simulink model "HIL_Testing_SW_amantest"  (Simulink 7.5)
settings: Solver=ode1  StartTime=0.0  StopTime=Inf  FixedStep=0.001  RelTol=1e-3
PostLoadFcn:
  | , if any(exist('dsrtsu_mdlpostloadfcn', 'file') == [2, 3, 6]), try dsrtsu_mdlpostloadfcn('Execute', bdroot); catch fprintf('Error in PostLoadFcn (dsrtsu_mdlpostloadfcn) for model "%s":\n %s\n', bdroot, lasterr); end, end,
undefined symbols (not defined in the file): CeBSER_Cnt_NumTempAxisPts, ChargeCord, ChargeCord_Control, ChargeToSOCCurr, ChrgCurrLim, CrntSens1Fine, CS_SOCSetPt, CyclerMaxChrgPwr, CyclerMaxDschrgPwr, deltaAhr, Drive_1, Drive_10, Drive_11, Drive_12, Drive_13, Drive_14, Drive_15, Drive_16, Drive_17, Drive_18, Drive_19, Drive_2, Drive_20, Drive_21, Drive_22, Drive_23, Drive_24, Drive_25, Drive_26, Drive_27, Drive_28, Drive_29, Drive_3, Drive_30, Drive_31, Drive_32, Drive_33, Drive_34, Drive_35, Drive_36, Drive_37, Drive_38, Drive_39, Drive_4, Drive_40, Drive_41, Drive_42, Drive_43, Drive_44, Drive_45, Drive_46, Drive_47, Drive_48, Drive_49, Drive_5, Drive_50, Drive_51, Drive_6, Drive_7, Drive_8 ... (+50)
libraries: simulink x129, rtican x50, rti2211sailib x5, rti2211serlib x5, rti2202miolib x3
(part 23 of 23)

== stateflow chart LionsHeart/FeaturePresentation/Down_to_Business/DriveProfile_ModeControl/Scirpt Test ==
  state SwitchProfile
    entry:
    Step=Step+1;
    IndicatorSF = 2;
    ProfileClassIndex=GetIndex(ProfileScheduleClass,Step);
  state Corvette
    entry:
    IndicatorSF=0;
    PowerCycle=0;
    du:
    PowerCycle=0;
  state End_Suite
    entry:
    EndStep=99
    IndicatorSF=2;
    ex: EndStep=0;
    IndicatorSF=2;
  state Acadia
    entry:
    IndicatorSF=0;
    PowerCycle=3;
    du:
    PowerCycle=3;
  state ATS
    entry:
    IndicatorSF=0;
    PowerCycle=1;
    du:
    PowerCycle=1;
  state PowerPulse_Discharge
    entry:
    Wait=0;
    IndicatorSF=5;
    Direction =2;
    du:
    Wait=Wait+sim_step_time;
  state start
    entry:
    SuiteStep=0;
    EndStep=0;
    IndicatorSF=2;
  state Return
  state OneHundredTen_V_Charge
    entry:
    IndicatorSF = 1;
    ChargeCurrSelect=0;
    during: ChargeCurrSelect=0;
  state RestTimer
    entry:
    IndicatorSF = 2;
    RestTime = 0;
    du:
    RestTime = RestTime+sim_step_time;
  state PowerPulse_Charge
    entry:
    IndicatorSF=5;
    Direction =1;
    Wait=0;
    du:
    Wait=Wait+sim_step_time;
  state Yukon
    entry:
    IndicatorSF=0;
    PowerCycle=51;
    du:
    PowerCycle=51;
  state TwoHundredTwenty_V_Charge
    entry:
    IndicatorSF = 1;
    ChargeCurrSelect=1;
    during: ChargeCurrSelect=1;
  state XTS
    entry:
    IndicatorSF=0;
    PowerCycle=50;
    du:
    PowerCycle=50;
  state Charge_To_SOC
    entry:
    IndicatorSF = 1;
    ChargeCurrSelect=2;
    during: ChargeCurrSelect=2;
  state Reset_SOC_and_Ahr
    entry:
    IndicatorSF = 2;
    ResetSOC=1;
    ResetWaitTime=0;
    during: ResetSOC=1;
    ResetWaitTime=ResetWaitTime+sim_step_time;
    exit: ResetSOC=0;
  state Determine_Charge_Type
    entry:
    IndicatorSF = 1;
    ProfileTypeIndex=GetIndex(ProfileScheduleType,Step);
  state Determine_Drive_Type
    entry:
    IndicatorSF = 0;
    ProfileTypeIndex=GetIndex(ProfileScheduleType,Step);
  state Determine_PowerPulse_Type
    entry:
    IndicatorSF = 1;
    ProfileTypeIndex=GetIndex(ProfileScheduleType,Step);
  state Verano
    entry:
    IndicatorSF=0;
    PowerCycle=49;
    du:
    PowerCycle=49;
  state Apply_SOC_Target
    entry:
    ProfileParameter = GetIndex(ProfileScheduleParameter,Step);
    SOCTarget = ProfileParameter/100;
  state Determine_Rest_Time
    entry:
    ProfileParameter = GetIndex(ProfileScheduleParameter,Step);
  state Apply_RestTimeIn
    entry:
    RestTimeTarget = RestTimeIn;
  state Apply_ProfileParameter
    entry:
    RestTimeTarget = ProfileParameter;
  state SwitchSuite
    entry:
    SuiteStep=SuiteStep+1;
    EndStep=2;
    Step=0;
    RepeatIndex = 0;
    IndicatorSF = 2;
    SuiteIndex=GetSuiteIndex(SuiteSchedule,SuiteStep);
    Suite = SuiteIndex;
  state PrimePack_Suite
    entry:
    ProfileScheduleClass = PrimePackClass;
    ProfileScheduleType = PrimePackType;
    ProfileScheduleParameter = PrimePackParameter;
  state Use_Profile_Builder
    entry:
    ProfileScheduleClass = ProfileScheduleClassIn;
    ProfileScheduleType= ProfileScheduleTypeIn;
    ProfileScheduleParameter = ProfileScheduleParameterIn;
    ProfileScheduleParameter2 = ProfileScheduleParameterIn2;
  state Drive_With_Pulses_Suite
    entry:
    ProfileScheduleClass = DrivesWithPulsesClass;
    ProfileScheduleType = DrivesWithPulsesType;
    ProfileScheduleParameter = DrivesWithPulsesParameter;
  state End_Test
    entry:
    IndicatorSF=2;
  state Drive_To_PIC
    entry:
    ProfileScheduleClass = DriveToPICClass;
    ProfileScheduleType = DriveToPICType;
    ProfileScheduleParameter = DriveToPICParameter;
  state Aztek
    entry:
    IndicatorSF=0;
    PowerCycle=2;
    du:
    PowerCycle=2;
  state Aura
    entry:
    IndicatorSF=0;
    PowerCycle=4;
    du:
    PowerCycle=4;
  state Bel_Air
    entry:
    IndicatorSF=0;
    PowerCycle=5;
    du:
    PowerCycle=5;
  state Cruze
    entry:
    IndicatorSF=0;
    PowerCycle=6;
    du:
    PowerCycle=6;
  state Camaro
    entry:
    IndicatorSF=0;
    PowerCycle=7;
    du:
    PowerCycle=7;
  state Apply_Volt_Target1
    entry:
    ProfileParameter = GetIndex(ProfileScheduleParameter,Step);
    VoltTarget = ProfileParameter;
  state Apply_Volt_Target2
    entry:
    ProfileParameter = GetIndex(ProfileScheduleParameter,Step);
    VoltTarget = ProfileParameter;
  state Reset_Run
    entry:
    IndicatorSF = 2;
    ResetTime = 0;
    ResetRun = 1;
    du:
    ResetRun=1;
    ResetTime = ResetTime+sim_step_time;
    exit:
    ResetRun=0;
    SetChamberT_ToBatTemp = 0;
  state Determine_Reset_Time
    entry:
    ProfileParameter = GetIndex(ProfileScheduleParameter,Step);
  state Apply_DefaultTime
    entry:
    ResetTarget = 150;
  state Apply_ParameterTime
    entry:
    ResetTarget = ProfileParameter;
  state Capacity_Test
    entry:
    IndicatorSF = 3;
    du:
    IndicatorSF = 3;
  state Caprice
    entry:
    IndicatorSF=0;
    PowerCycle=8;
    du:
    PowerCycle=8;
  state Colorado
    entry:
    IndicatorSF=0;
    PowerCycle=9;
    du:
    PowerCycle=9;
  state CTSv
    entry:
    IndicatorSF=0;
    PowerCycle=10;
    du:
    PowerCycle=10;
  state Cobalt
    entry:
    IndicatorSF=0;
    PowerCycle=11;
    du:
    PowerCycle=11;
  state TimerForContactorstoClose
    entry:
    WTime=0;
    du:
    WTime=WTime+sim_step_time;
  state DTS
    entry:
    IndicatorSF=0;
    PowerCycle=12;
    du:
    PowerCycle=12;
  state El_Camino
    entry:
    IndicatorSF=0;
    PowerCycle=13;
    du:
    PowerCycle=13;
  state Equinox
    entry:
    IndicatorSF=0;
    PowerCycle=14;
    du:
    PowerCycle=14;
  state Encore
    entry:
    IndicatorSF=0;
    PowerCycle=15;
    du:
    PowerCycle=15;
  state Enclave
    entry:
    IndicatorSF=0;
    PowerCycle=16;
    du:
    PowerCycle=16;
  state OCV_Test
    entry:
    IndicatorSF = 6;
    du:
    IndicatorSF = 6;
  state ELR
    entry:
    IndicatorSF=0;
    PowerCycle=17;
    du:
    PowerCycle=17;
  state El_Dorado
    entry:
    IndicatorSF=0;
    PowerCycle=18;
    du:
    PowerCycle=18;
  state HHR
    entry:
    IndicatorSF=0;
    PowerCycle=19;
    du:
    PowerCycle=19;
  state Impala
    entry:
    IndicatorSF=0;
    PowerCycle=20;
    du:
    PowerCycle=20;
  state Lacrosse
    entry:
    IndicatorSF=0;
    PowerCycle=21;
    du:
    PowerCycle=21;
  state MontiCarlo
    entry:
    IndicatorSF=0;
    PowerCycle=22;
    du:
    PowerCycle=22;
  state Malibu
    entry:
    IndicatorSF=0;
    PowerCycle=23;
    du:
    PowerCycle=23;
  state Montana
    entry:
    IndicatorSF=0;
    PowerCycle=24;
    du:
    PowerCycle=24;
  state Nova
    entry:
    IndicatorSF=0;
    PowerCycle=25;
    du:
    PowerCycle=25;
  state Determine_Drive_Start
    entry:
    IndicatorSF = 0;
    StartTime=GetIndex(ProfileScheduleParameter,Step);
  state Determine_Drive_End
    entry:
    IndicatorSF = 0;
    EndTime=GetIndex(ProfileScheduleParameter2,Step);
  state Chevelle
    entry:
    IndicatorSF=0;
    PowerCycle=26;
    du:
    PowerCycle=26;
  state Idle_ConstPower
    entry:
    IndicatorSF =7;
    Wait =0;
    du:
    IndicatorSF = 7;
    Wait = Wait +sim_step_time;
  state Determine_Idle_ConstPower_Time
    entry:
    ProfileParameter = GetIndex(ProfileScheduleParameter,Step);
    IdleTime=ProfileParameter;
    Idle_Type = 1;
  state Determine_IdlePower
    entry:
    ProfileParameter = GetIndex(ProfileScheduleParameter2,Step);
    PowerReq=ProfileParameter;
  state Chevette
    entry:
    IndicatorSF=0;
    PowerCycle=27;
    du:
    PowerCycle=27;
  state Corvair
    entry:
    IndicatorSF=0;
    PowerCycle=28;
    du:
    PowerCycle=28;
  state GrandPrix
    entry:
    IndicatorSF=0;
    PowerCycle=29;
    du:
    PowerCycle=29;
  state G6
    entry:
    IndicatorSF=0;
    PowerCycle=30;
    du:
    PowerCycle=30;
  state Determine_RaterPulse_Type
    entry:
    IndicatorSF = 2;
    ProfileTypeIndex=GetIndex(ProfileScheduleType,Step);
  state RatePulse_Discharge
    entry:
    Wait=0;
    IndicatorSF=8;
    Direction =2;
    du:
    Wait=Wait+sim_step_time;
  state RatePulse_Charge
    entry:
    IndicatorSF=8;
    Direction =1;
    Wait=0;
    du:
    Wait=Wait+sim_step_time;
  state Determine_CurrentLimit
    entry:
    ProfileParameter = GetIndex(ProfileScheduleParameter,Step);
    CurrLim=ProfileParameter;
  state Determine_Rate
    entry:
    ProfileParameter = GetIndex(ProfileScheduleParameter2,Step);
    Rate=ProfileParameter;
  state Increment_Test
    entry:
    IndicatorSF = 9;
    du:
    IndicatorSF = 9;
  state G8
    entry:
    IndicatorSF=0;
    PowerCycle=31;
    du:
    PowerCycle=31;
  state Outlook
    entry:
    IndicatorSF=0;
    PowerCycle=32;
    du:
    PowerCycle=32;
  state Canyon
    entry:
    IndicatorSF=0;
    PowerCycle=33;
    du:
    PowerCycle=33;
  state Firebird
    entry:
    IndicatorSF=0;
    PowerCycle=34;
    du:
    PowerCycle=34;
  state Regal
    entry:
    IndicatorSF=0;
    PowerCycle=35;
    du:
    PowerCycle=35;
  state Silverado
    entry:
    IndicatorSF=0;
    PowerCycle=36;
    du:
    PowerCycle=36;
  state Sierra
    entry:
    IndicatorSF=0;
    PowerCycle=37;
    du:
    PowerCycle=37;
  state Sonic
    entry:
    IndicatorSF=0;
    PowerCycle=38;
    du:
    PowerCycle=38;
  state Spark
    entry:
    IndicatorSF=0;
    PowerCycle=39;
    du:
    PowerCycle=39;
  state Sky
    entry:
    IndicatorSF=0;
    PowerCycle=40;
    du:
    PowerCycle=40;
  state Solstice
    entry:
    IndicatorSF=0;
    PowerCycle=41;
    du:
    PowerCycle=41;
  state SRX
    entry:
    IndicatorSF=0;
    PowerCycle=42;
    du:
    PowerCycle=42;
  state Escalade
    entry:
    IndicatorSF=0;
    PowerCycle=43;
    du:
    PowerCycle=43;
  state Terrain
    entry:
    IndicatorSF=0;
    PowerCycle=44;
    du:
    PowerCycle=44;
  state Torrent
    entry:
    IndicatorSF=0;
    PowerCycle=45;
    du:
    PowerCycle=45;
  state TransAm
    entry:
    IndicatorSF=0;
    PowerCycle=46;
    du:
    PowerCycle=46;
  state Traverse
    entry:
    IndicatorSF=0;
    PowerCycle=47;
    du:
    PowerCycle=47;
  state Tahoe
    entry:
    IndicatorSF=0;
    PowerCycle=48;
    du:
    PowerCycle=48;
  state Determine_SetChamberT_ToBatTemp
    entry:
    ProfileParameter = GetIndex(ProfileScheduleParameter2,Step);
    SetChamberT_ToBatTemp = ProfileParameter;
  state Apply_SetChamberT_ToBatTemp
    entry:
    SetChamberT_ToBatTemp = 1;
  state Apply_DontSetChamberT_ToBatTemp
    entry:
    SetChamberT_ToBatTemp = 0;
  state Idle_ConstCurrent
    entry:
    IndicatorSF =7;
    Wait =0;
    du:
    IndicatorSF = 7;
    Wait = Wait +sim_step_time;
  state Determine_Idle_ConstCurrent_Time
    entry:
    ProfileParameter = GetIndex(ProfileScheduleParameter,Step);
    IdleTime=ProfileParameter;
    Idle_Type = 2;
  state Determine_IdleCurrent
    entry:
    ProfileParameter = GetIndex(ProfileScheduleParameter2,Step);
    CurrentReq=ProfileParameter;
  state Determine_Idle_Type
    entry:
    IndicatorSF = 1;
    ProfileTypeIndex=GetIndex(ProfileScheduleType,Step);
  state Repeat
    entry:
    IndicatorSF = 2;
    RepeatCount = GetIndex(ProfileScheduleParameter,Step);
    RepeatStep
  state RepeatEnd
    entry:
    IndicatorSF = 2;
    RepeatIndex = 0;
    Step=Step+1;
  state RepeatJumpLoop
    entry:
    IndicatorSF = 2;
    Jumps = GetIndex(ProfileScheduleParameter2,Step);
    Jumps = Jumps + 1;
    during:
    RepeatIndex = RepeatIndex+1;
    Step=1;
    RepeatStep
  SwitchProfile -> Determine_Charge_Type [order 2] : [ProfileClassIndex == 1]
  Return -> (junction 900) [order 1] : [(Run==1) && (SkipStep==0)]
  Corvette -> Return [order 2] : [(LoopTime>= ProfileEndTime) && (LoopTime>0)]
  PowerPulse_Discharge -> Return [order 2] : [(PulseStep>= 2) && (Wait>1)]
  ATS -> Return [order 2] : [(LoopTime>= ProfileEndTime) && (LoopTime>0)]
  Determine_Charge_Type -> Apply_Volt_Target2 [order 2] : [ProfileTypeIndex==2]
  (default) -> start
  Corvette -> Return [order 1] : [Run==0]
  PowerPulse_Discharge -> Return [order 1] : [Run==0]
  ATS -> Return [order 1] : [Run==0]
  start -> SwitchSuite : [ManualMode==0 && Run == 1]
  Reset_SOC_and_Ahr -> Return [order 2] : [ResetWaitTime>=2]
  End_Suite -> start [order 2] : [Run==0]
  Determine_Drive_End -> Yukon [order 52] : [ProfileTypeIndex==52]
  OneHundredTen_V_Charge -> Return [order 2] : [ChargeStep>=99]
  RestTimer -> Return [order 2] : [RestTime>=RestTimeTarget]
  Determine_Drive_End -> Corvette [order 1] : [ProfileTypeIndex == 1]
  Reset_SOC_and_Ahr -> Return [order 1] : [Run==0]
  Determine_Drive_End -> Acadia [order 4] : [ProfileTypeIndex == 4]
  RestTimer -> Return [order 1] : [Run==0]
  Acadia -> Return [order 1] : [Run==0]
  Acadia -> Return [order 2] : [(LoopTime>= ProfileEndTime) && (LoopTime>0)]
  Determine_Charge_Type -> Apply_SOC_Target [order 3] : [ProfileTypeIndex==3]
  Determine_Charge_Type -> Apply_Volt_Target1 [order 1] : [ProfileTypeIndex==1]
  PowerPulse_Charge -> Return [order 2] : [(PulseStep>= 2) && (Wait>1)]
  Determine_Drive_End -> XTS [order 51] : [ProfileTypeIndex==51]
  SwitchProfile -> End_Suite [order 13] : [ProfileClassIndex==0]
  PowerPulse_Charge -> Return [order 1] : [Run==0]
  TwoHundredTwenty_V_Charge -> Return [order 2] : [ChargeStep>=99]
  TwoHundredTwenty_V_Charge -> Return [order 1] : [Run==0]
  Determine_Drive_End -> Tahoe [order 49] : [ProfileTypeIndex==49]
  Determine_Drive_End -> Traverse [order 48] : [ProfileTypeIndex==48]
  Determine_Drive_End -> ATS [order 2] : [ProfileTypeIndex == 2]
  SwitchProfile -> start [order 1] : [Run==0]
  OneHundredTen_V_Charge -> Return [order 3] : [SkipStep==1]
  TwoHundredTwenty_V_Charge -> Return [order 3] : [SkipStep==1]
  Determine_Drive_End -> TransAm [order 47] : [ProfileTypeIndex==47]
  RestTimer -> Return [order 3] : [SkipStep==1]
  Corvette -> Return [order 3] : [SkipStep==1]
  ATS -> Return [order 3] : [SkipStep==1]
  Acadia -> Return [order 3] : [SkipStep==1]
  PowerPulse_Charge -> Return [order 3] : [SkipStep==1]
  Determine_Drive_End -> Torrent [order 46] : [ProfileTypeIndex==46]
  Determine_Drive_End -> Terrain [order 45] : [ProfileTypeIndex==45]
  Determine_Drive_End -> Escalade [order 44] : [ProfileTypeIndex==44]
  Reset_SOC_and_Ahr -> Return [order 3] : [SkipStep==1]
  Charge_To_SOC -> Return [order 1] : [ChargeStep>=99]
  Charge_To_SOC -> Return [order 2] : [Run==0]
  Charge_To_SOC -> Return [order 3] : [SkipStep==1]
  Determine_Drive_End -> Verano [order 50] : [ProfileTypeIndex==50]
  SwitchProfile -> Determine_Drive_Type [order 5] : [ProfileClassIndex == 2]
  Determine_PowerPulse_Type -> PowerPulse_Discharge [order 1] : [ProfileTypeIndex == 1]
  Determine_PowerPulse_Type -> PowerPulse_Charge [order 2] : [ProfileTypeIndex == 2]
  SwitchProfile -> Determine_PowerPulse_Type [order 6] : [ProfileClassIndex == 3]
  SwitchProfile -> Determine_Rest_Time [order 10] : [ProfileClassIndex == 5]
  SwitchProfile -> Reset_SOC_and_Ahr [order 8] : [ProfileClassIndex == 4]
  Determine_Drive_End -> Spark [order 40] : [ProfileTypeIndex==40]
  Determine_Drive_End -> Sonic [order 39] : [ProfileTypeIndex==39]
  Determine_Drive_End -> Sierra [order 38] : [ProfileTypeIndex==38]
  Determine_Drive_End -> Sky [order 41] : [ProfileTypeIndex==41]
  Apply_SOC_Target -> Charge_To_SOC [order 2]
  Determine_Rest_Time -> Apply_RestTimeIn [order 1] : [ProfileParameter == 0]
  Apply_RestTimeIn -> RestTimer
  Determine_Rest_Time -> Apply_ProfileParameter [order 2] : [ProfileParameter != 0]
  Apply_ProfileParameter -> RestTimer
  SwitchSuite -> PrimePack_Suite [order 1] : [SuiteIndex == 1]
  SwitchSuite -> Use_Profile_Builder [order 4] : [SuiteIndex == 10]
  SwitchSuite -> Drive_With_Pulses_Suite [order 2] : [SuiteIndex == 2]
  PrimePack_Suite -> SwitchProfile
  Drive_With_Pulses_Suite -> SwitchProfile
  Use_Profile_Builder -> SwitchProfile
  End_Suite -> SwitchSuite [order 1] : after(1000,tick) [(Run==1) && (SkipStep==0)]
  SwitchSuite -> End_Test [order 5] : [SuiteIndex == 0]
  End_Test -> start : [Run == 0]
  SwitchSuite -> Drive_To_PIC [order 3] : [SuiteIndex == 3]
  Drive_To_PIC -> SwitchProfile
  PowerPulse_Discharge -> Return [order 3] : [SkipStep==1]
  (junction 900) -> Use_Profile_Builder [order 2] : [SuiteIndex == 10]
  (junction 900) -> SwitchProfile [order 1] : [SuiteIndex != 10]
  Aztek -> Return [order 2] : [(LoopTime>= ProfileEndTime) && (LoopTime>0)]
  Aztek -> Return [order 1] : [Run==0]
  Aztek -> Return [order 3] : [SkipStep==1]
  Determine_Drive_End -> Aztek [order 3] : [ProfileTypeIndex == 3]
  Aura -> Return [order 1] : [Run==0]
  Aura -> Return [order 2] : [(LoopTime>= ProfileEndTime) && (LoopTime>0)]
  Aura -> Return [order 3] : [SkipStep==1]
  Bel_Air -> Return [order 1] : [Run==0]
  Bel_Air -> Return [order 2] : [(LoopTime>= ProfileEndTime) && (LoopTime>0)]
  Bel_Air -> Return [order 3] : [SkipStep==1]
  Cruze -> Return [order 1] : [Run==0]
  Cruze -> Return [order 2] : [(LoopTime>= ProfileEndTime) && (LoopTime>0)]
  Cruze -> Return [order 3] : [SkipStep==1]
  Camaro -> Return [order 1] : [Run==0]
  Camaro -> Return [order 2] : [(LoopTime>= ProfileEndTime) && (LoopTime>0)]
  Camaro -> Return [order 3] : [SkipStep==1]
  Camaro -> Return [order 4] : [(EnblSOCTerm==1) && (SOC<(SOCDeplete))]
  Cruze -> Return [order 4] : [(EnblSOCTerm==1) && (SOC<(SOCDeplete))]
  Bel_Air -> Return [order 4] : [(EnblSOCTerm==1) && (SOC<(SOCDeplete))]
  Determine_Drive_End -> Aura [order 5] : [ProfileTypeIndex == 5]
  Determine_Drive_End -> Bel_Air [order 6] : [ProfileTypeIndex == 6]
  Determine_Drive_End -> Cruze [order 7] : [ProfileTypeIndex == 7]
  Determine_Drive_End -> Camaro [order 8] : [ProfileTypeIndex == 8]
  Aura -> Return [order 4] : [(EnblSOCTerm==1) && (SOC<(SOCDeplete/100))]
  Apply_SOC_Target -> Return [order 1] : [(SOCTarget > 100) || (SOCTarget < 0)]
  OneHundredTen_V_Charge -> Return [order 1] : [Run==0]
  Corvette -> Return [order 4] : [(EnblSOCTerm==1) && (SOC<(SOCDeplete))]
  ATS -> Return [order 4] : [(EnblSOCTerm==1) && (SOC<(SOCDeplete))]
  Aztek -> Return [order 4] : [(EnblSOCTerm==1) && (SOC<(SOCDeplete))]
  Acadia -> Return [order 4] : [(EnblSOCTerm==1) && (SOC<(SOCDeplete))]
  Apply_Volt_Target1 -> OneHundredTen_V_Charge
  Determine_Drive_End -> Lacrosse [order 23] : [ProfileTypeIndex == 22]
  Apply_Volt_Target2 -> TwoHundredTwenty_V_Charge
  Determine_Drive_End -> Impala [order 21] : [ProfileTypeIndex == 21]
  Reset_Run -> TimerForContactorstoClose [order 1] : [ResetTime>=ResetTarget]
  Reset_Run -> Return [order 2] : [Run==0]
  Reset_Run -> Return [order 3] : [SkipStep==1]
  Determine_Reset_Time -> Apply_DefaultTime [order 1] : [ProfileParameter == 0]
  Determine_Reset_Time -> Apply_ParameterTime [order 2] : [ProfileParameter != 0]
  Apply_DefaultTime -> Determine_SetChamberT_ToBatTemp
  Apply_ParameterTime -> Determine_SetChamberT_ToBatTemp
  SwitchProfile -> Determine_Reset_Time [order 12] : [ProfileClassIndex ==6]
  SwitchProfile -> Capacity_Test [order 7] : [ProfileClassIndex==7]
  Capacity_Test -> Return [order 3] : [SkipStep==1]
  Capacity_Test -> Return [order 2] : [CapStep==99]
  Capacity_Test -> Return [order 1] : [Run==0]
  Determine_Drive_End -> Caprice [order 9] : [ProfileTypeIndex == 9]
  Caprice -> Return [order 1] : [Run==0]
  Caprice -> Return [order 2] : [(LoopTime>= ProfileEndTime) && (LoopTime>0)]
  Caprice -> Return [order 3] : [SkipStep==1]
  Caprice -> Return [order 4] : [(EnblSOCTerm==1) && (SOC<(SOCDeplete))]
  Determine_Drive_End -> Colorado [order 10] : [ProfileTypeIndex == 10]
  Determine_Drive_End -> CTSv [order 11] : [ProfileTypeIndex == 11]
  Colorado -> Return [order 1] : [Run==0]
  Colorado -> Return [order 2] : [(LoopTime>= ProfileEndTime) && (LoopTime>0)]
  Colorado -> Return [order 3] : [SkipStep==1]
  Colorado -> Return [order 4] : [(EnblSOCTerm==1) && (SOC<(SOCDeplete))]
  CTSv -> Return [order 1] : [Run==0]
  CTSv -> Return [order 2] : [(LoopTime>= ProfileEndTime) && (LoopTime>0)]
  CTSv -> Return [order 3] : [SkipStep==1]
  CTSv -> Return [order 4] : [(EnblSOCTerm==1) && (SOC<(SOCDeplete))]
  Determine_Drive_End -> Cobalt [order 12] : [ProfileTypeIndex == 12]
  Cobalt -> Return [order 1] : [Run==0]
  Cobalt -> Return [order 2] : [(LoopTime>= ProfileEndTime) && (LoopTime>0)]
  Cobalt -> Return [order 3] : [SkipStep==1]
  Cobalt -> Return [order 4] : [(EnblSOCTerm==1) && (SOC<(SOCDeplete/100))]
  TimerForContactorstoClose -> Return [order 1] : [WTime>10]
  TimerForContactorstoClose -> Return [order 2] : [Run==0]
  TimerForContactorstoClose -> Return [order 3] : [SkipStep==1]
  Determine_Drive_End -> DTS [order 13] : [ProfileTypeIndex == 13]
  DTS -> Return [order 1] : [Run==0]
  DTS -> Return [order 2] : [(LoopTime>= ProfileEndTime) && (LoopTime>0)]
  DTS -> Return [order 3] : [SkipStep==1]
  DTS -> Return [order 4] : [(EnblSOCTerm==1) && (SOC<(SOCDeplete))]
  El_Camino -> Return [order 1] : [Run==0]
  El_Camino -> Return [order 2] : [(LoopTime>= ProfileEndTime) && (LoopTime>0)]
  El_Camino -> Return [order 3] : [SkipStep==1]
  El_Camino -> Return [order 4] : [(EnblSOCTerm==1) && (SOC<(SOCDeplete))]
  Determine_Drive_End -> El_Camino [order 14] : [ProfileTypeIndex == 14]
  Equinox -> Return [order 1] : [Run==0]
  Equinox -> Return [order 2] : [(LoopTime>= ProfileEndTime) && (LoopTime>0)]
  Equinox -> Return [order 3] : [SkipStep==1]
  Equinox -> Return [order 4] : [(EnblSOCTerm==1) && (SOC<(SOCDeplete))]
  Determine_Drive_End -> Equinox [order 15] : [ProfileTypeIndex == 15]
  Encore -> Return [order 1] : [Run==0]
  Encore -> Return [order 2] : [(LoopTime>= ProfileEndTime) && (LoopTime>0)]
  Encore -> Return [order 3] : [SkipStep==1]
  Encore -> Return [order 4] : [(EnblSOCTerm==1) && (SOC<(SOCDeplete))]
  Enclave -> Return [order 1] : [Run==0]
  Enclave -> Return [order 2] : [(LoopTime>= ProfileEndTime) && (LoopTime>0)]
  Enclave -> Return [order 3] : [SkipStep==1]
  Enclave -> Return [order 4] : [(EnblSOCTerm==1) && (SOC<(SOCDeplete))]
  Determine_Drive_End -> Encore [order 17] : [ProfileTypeIndex == 16]
  Determine_Drive_End -> Enclave [order 16] : [ProfileTypeIndex == 17]
  OCV_Test -> Return [order 3] : [SkipStep==1]
  OCV_Test -> Return [order 2] : [OCVStep==99]
  OCV_Test -> Return [order 1] : [Run==0]
  SwitchProfile -> RepeatJumpLoop [order 4] : [RepeatIndex !=0 && ProfileClassIndex==100]
  ELR -> Return [order 1] : [Run==0]
  ELR -> Return [order 2] : [(LoopTime>= ProfileEndTime) && (LoopTime>0)]
  ELR -> Return [order 3] : [SkipStep==1]
  ELR -> Return [order 4] : [(EnblSOCTerm==1) && (SOC<(SOCDeplete))]
  El_Dorado -> Return [order 1] : [Run==0]
  El_Dorado -> Return [order 2] : [(LoopTime>= ProfileEndTime) && (LoopTime>0)]
  El_Dorado -> Return [order 3] : [SkipStep==1]
  El_Dorado -> Return [order 5] : [(EnblSOCTerm==1) && (SOC<(SOCDeplete))]
  HHR -> Return [order 1] : [Run==0]
  HHR -> Return [order 2] : [(LoopTime>= ProfileEndTime) && (LoopTime>0)]
  HHR -> Return [order 4] : [SkipStep==1]
  HHR -> Return [order 5] : [(EnblSOCTerm==1) && (SOC<(SOCDeplete))]
  Impala -> Return [order 1] : [Run==0]
  Impala -> Return [order 3] : [(LoopTime>= ProfileEndTime) && (LoopTime>0)]
  Impala -> Return [order 4] : [SkipStep==1]
  Impala -> Return [order 5] : [(EnblSOCTerm==1) && (SOC<(SOCDeplete))]
  Lacrosse -> Return [order 2] : [(LoopTime>= ProfileEndTime) && (LoopTime>0)]
  Lacrosse -> Return [order 3] : [SkipStep==1]
  Lacrosse -> Return [order 4] : [(EnblSOCTerm==1) && (SOC<(SOCDeplete))]
  Lacrosse -> Return [order 1] : [Run==0]
  Determine_Drive_End -> ELR [order 18] : [ProfileTypeIndex == 18]
  Determine_Drive_End -> El_Dorado [order 19] : [ProfileTypeIndex == 19]
  Determine_Drive_End -> HHR [order 20] : [ProfileTypeIndex == 20]
  MontiCarlo -> Return [order 2] : [(LoopTime>= ProfileEndTime) && (LoopTime>0)]
  MontiCarlo -> Return [order 4] : [SkipStep==1]
  MontiCarlo -> Return [order 5] : [(EnblSOCTerm==1) && (SOC<(SOCDeplete))]
  MontiCarlo -> Return [order 1] : [Run==0]
  Malibu -> Return [order 2] : [(LoopTime>= ProfileEndTime) && (LoopTime>0)]
  Malibu -> Return [order 3] : [SkipStep==1]
  Malibu -> Return [order 4] : [(EnblSOCTerm==1) && (SOC<(SOCDeplete))]
  Malibu -> Return [order 1] : [Run==0]
  Montana -> Return [order 2] : [(LoopTime>= ProfileEndTime) && (LoopTime>0)]
  Montana -> Return [order 3] : [SkipStep==1]
  Montana -> Return [order 4] : [(EnblSOCTerm==1) && (SOC<(SOCDeplete))]
  Montana -> Return [order 1] : [Run==0]
  Nova -> Return [order 2] : [(LoopTime>= ProfileEndTime) && (LoopTime>0)]
  Nova -> Return [order 3] : [SkipStep==1]
  Nova -> Return [order 4] : [(EnblSOCTerm==1) && (SOC<(SOCDeplete))]
  RatePulse_Charge -> Return [order 4] : [(EnblSOCTerm==1) && (SOC<(SOCDeplete))]
  Determine_Drive_End -> MontiCarlo [order 22] : [ProfileTypeIndex==23]
  Determine_Drive_End -> Malibu [order 29] : [ProfileTypeIndex==24]
  Determine_Drive_End -> Montana [order 31] : [ProfileTypeIndex==25]
  Determine_Drive_End -> Nova [order 30] : [ProfileTypeIndex==26]
  Corvette -> Return [order 5] : [SwitchMode==1]
  ATS -> Return [order 5] : [SwitchMode==1]
  Aztek -> Return [order 5] : [SwitchMode==1]
  Acadia -> Return [order 5] : [SwitchMode==1]
  Aura -> Return [order 5] : [SwitchMode==1]
  Bel_Air -> Return [order 5] : [SwitchMode==1]
  Cruze -> Return [order 5] : [SwitchMode==1]
  Camaro -> Return [order 5] : [SwitchMode==1]
  Caprice -> Return [order 5] : [SwitchMode==1]
  Colorado -> Return [order 5] : [SwitchMode==1]
  CTSv -> Return [order 5] : [SwitchMode==1]
  Cobalt -> Return [order 5] : [SwitchMode==1]
  DTS -> Return [order 5] : [SwitchMode==1]
  El_Camino -> Return [order 5] : [SwitchMode==1]
  Equinox -> Return [order 5] : [SwitchMode==1]
  Encore -> Return [order 5] : [SwitchMode==1]
  Enclave -> Return [order 5] : [SwitchMode==1]
  Determine_Drive_Type -> Determine_Drive_Start
  Determine_Drive_Start -> Determine_Drive_End
  Chevelle -> Return [order 1] : [Run==0]
  Chevelle -> Return [order 2] : [(LoopTime>= ProfileEndTime) && (LoopTime>0)]
  Chevelle -> Return [order 3] : [SkipStep==1]
  Nova -> Return [order 1] : [Run==0]
  Chevelle -> Return [order 4] : [(EnblSOCTerm==1) && (SOC<(SOCDeplete))]
  Determine_Drive_End -> Chevelle [order 24] : [ProfileTypeIndex==27]
  Idle_ConstPower -> Return [order 4] : [SkipStep==1]
  Idle_ConstPower -> Return [order 3] : [(IdleStep==99) && (Wait>1)]
  Idle_ConstPower -> Return [order 1] : [Run==0]
  Apply_DontSetChamberT_ToBatTemp -> Reset_Run
  Determine_Idle_ConstPower_Time -> Determine_IdlePower [order 1] : [IdleTime!=0]
  Determine_Idle_ConstPower_Time -> Return [order 2] : [IdleTime==0]
  Idle_ConstPower -> Return [order 2] : [FA!=0]
  OneHundredTen_V_Charge -> Return [order 4] : [FA!=0]
  TwoHundredTwenty_V_Charge -> Return [order 4] : [FA!=0]
  Determine_Drive_End -> SRX [order 43] : [ProfileTypeIndex==43]
  Determine_Drive_End -> Solstice [order 42] : [ProfileTypeIndex==42]
  Charge_To_SOC -> Return [order 4] : [FA!=0]
  Determine_Drive_End -> Silverado [order 37] : [ProfileTypeIndex==37]
  Corvette -> Return [order 6] : [FA!=0]
  ATS -> Return [order 6] : [FA!=0]
  Aztek -> Return [order 6] : [FA!=0]
  Acadia -> Return [order 6] : [FA!=0]
  Aura -> Return [order 6] : [FA!=0]
  Bel_Air -> Return [order 6] : [FA!=0]
  Cruze -> Return [order 6] : [FA!=0]
  Camaro -> Return [order 6] : [FA!=0]
  Caprice -> Return [order 6] : [FA!=0]
  Colorado -> Return [order 6] : [FA!=0]
  CTSv -> Return [order 6] : [FA!=0]
  Cobalt -> Return [order 6] : [FA!=0]
  DTS -> Return [order 6] : [FA!=0]
  El_Camino -> Return [order 6] : [FA!=0]
  Equinox -> Return [order 6] : [FA!=0]
  Encore -> Return [order 6] : [FA!=0]
  Enclave -> Return [order 6] : [FA!=0]
  ELR -> Return [order 6] : [FA!=0]
  HHR -> Return [order 6] : [FA!=0]
  Impala -> Return [order 6] : [FA!=0]
  Lacrosse -> Return [order 6] : [FA!=0]
  MontiCarlo -> Return [order 6] : [FA!=0]
  Malibu -> Return [order 5] : [FA!=0]
  Montana -> Return [order 5] : [FA!=0]
  Nova -> Return [order 5] : [FA!=0]
  Chevelle -> Return [order 5] : [FA!=0]
  PowerPulse_Discharge -> Return [order 4] : [FA!=0]
  PowerPulse_Charge -> Return [order 4] : [FA!=0]
  Reset_SOC_and_Ahr -> Return [order 4] : [FA!=0]
  RestTimer -> Return [order 4] : [FA!=0]
  Capacity_Test -> Return [order 4] : [FA!=0]
  OCV_Test -> Return [order 4] : [FA!=0]
  Determine_IdlePower -> Idle_ConstPower [order 1] : [(PowerReq!=0) || (ManualIdle==1)]
  Determine_IdlePower -> Return [order 2] : [(PowerReq)==0 && (ManualIdle!=1)]
  G6 -> Return [order 5] : [FA!=0]
  Chevette -> Return [order 1] : [Run==0]
  Chevette -> Return [order 2] : [(LoopTime>= ProfileEndTime) && (LoopTime>0)]
  Chevette -> Return [order 3] : [SkipStep==1]
  Chevette -> Return [order 4] : [(EnblSOCTerm==1) && (SOC<(SOCDeplete))]
  MontiCarlo -> Return [order 3] : [SwitchMode==1]
  Determine_Drive_End -> Chevette [order 27] : [ProfileTypeIndex==28]
  Chevette -> Return [order 6] : [FA!=0]
  Determine_Drive_End -> G6 [order 25] : [ProfileTypeIndex==31]
  Corvair -> Return [order 1] : [Run==0]
  Corvair -> Return [order 2] : [(LoopTime>= ProfileEndTime) && (LoopTime>0)]
  Corvair -> Return [order 3] : [SkipStep==1]
  Corvair -> Return [order 4] : [(EnblSOCTerm==1) && (SOC<(SOCDeplete))]
  RatePulse_Discharge -> Return [order 5] : [(EnblSOCTerm==1) && (SOC<(SOCDeplete))]
  Determine_Drive_End -> Corvair [order 28] : [ProfileTypeIndex==29]
  Corvair -> Return [order 6] : [FA!=0]
  Corvair -> Return [order 5] : [SwitchMode==1]
  GrandPrix -> Return [order 1] : [Run==0]
  GrandPrix -> Return [order 2] : [(LoopTime>= ProfileEndTime) && (LoopTime>0)]
  GrandPrix -> Return [order 3] : [SkipStep==1]
  GrandPrix -> Return [order 4] : [(EnblSOCTerm==1) && (SOC<(SOCDeplete))]
  Chevette -> Return [order 5] : [SwitchMode==1]
  Determine_Drive_End -> GrandPrix [order 26] : [ProfileTypeIndex==30]
  GrandPrix -> Return [order 5] : [FA!=0]
  G6 -> Return [order 4] : [(EnblSOCTerm==1) && (SOC<(SOCDeplete))]
  G6 -> Return [order 1] : [Run==0]
  G6 -> Return [order 2] : [(LoopTime>= ProfileEndTime) && (LoopTime>0)]
  G6 -> Return [order 3] : [SkipStep==1]
  Determine_CurrentLimit -> Determine_Rate [order 1] : [CurrLim!=0]
  Determine_Rate -> Determine_RaterPulse_Type [order 1] : [Rate!=0]
  Determine_CurrentLimit -> Return [order 2] : [CurrLim==0]
  Determine_Rate -> Return [order 2] : [Rate==0]
  Determine_RaterPulse_Type -> RatePulse_Discharge [order 1] : [ProfileTypeIndex==1]
  Determine_RaterPulse_Type -> RatePulse_Charge [order 2] : [ProfileTypeIndex==2]
  RatePulse_Discharge -> Return [order 2] : [(RateStep== 2) && (Wait>1)]
  RatePulse_Discharge -> Return [order 1] : [Run==0]
  RatePulse_Discharge -> Return [order 3] : [SkipStep==1]
  RatePulse_Discharge -> Return [order 4] : [FA!=0]
  RatePulse_Charge -> Return [order 5] : [FA!=0]
  RatePulse_Charge -> Return [order 2] : [(RateStep== 2) && (Wait>1)]
  RatePulse_Charge -> Return [order 1] : [Run==0]
  RatePulse_Charge -> Return [order 3] : [SkipStep==1]
  Apply_SetChamberT_ToBatTemp -> Reset_Run
  Determine_SetChamberT_ToBatTemp -> Apply_DontSetChamberT_ToBatTemp [order 2] : [SetChamberT_ToBatTemp == 0]
  Increment_Test -> Return [order 1] : [Run==0]
  Increment_Test -> Return [order 2] : [IncrementStep==99]
  Increment_Test -> Return [order 3] : [SkipStep ==1]
  Increment_Test -> Return [order 4] : [FA!=0]
  Determine_Drive_End -> G8 [order 32] : [ProfileTypeIndex==32]
  Determine_Drive_End -> Outlook [order 33] : [ProfileTypeIndex==33]
  Determine_Drive_End -> Canyon [order 34] : [ProfileTypeIndex==34]
  Determine_Drive_End -> Firebird [order 35] : [ProfileTypeIndex==35]
  Determine_Drive_End -> Regal [order 36] : [ProfileTypeIndex==36]
  G8 -> Return [order 5] : [FA!=0]
  Lacrosse -> Return [order 5] : [SwitchMode==1]
  G8 -> Return [order 4] : [(EnblSOCTerm==1) && (SOC<(SOCDeplete))]
  G8 -> Return [order 1] : [Run==0]
  G8 -> Return [order 2] : [(LoopTime>= ProfileEndTime) && (LoopTime>0)]
  G8 -> Return [order 3] : [SkipStep==1]
  Outlook -> Return [order 5] : [FA!=0]
  Impala -> Return [order 2] : [SwitchMode==1]
  Outlook -> Return [order 4] : [(EnblSOCTerm==1) && (SOC<(SOCDeplete))]
  Outlook -> Return [order 1] : [Run==0]
  Outlook -> Return [order 2] : [(LoopTime>= ProfileEndTime) && (LoopTime>0)]
  Outlook -> Return [order 3] : [SkipStep==1]
  Canyon -> Return [order 5] : [FA!=0]
  HHR -> Return [order 3] : [SwitchMode==1]
  Canyon -> Return [order 4] : [(EnblSOCTerm==1) && (SOC<(SOCDeplete))]
  Canyon -> Return [order 1] : [Run==0]
  Canyon -> Return [order 2] : [(LoopTime>= ProfileEndTime) && (LoopTime>0)]
  Canyon -> Return [order 3] : [SkipStep==1]
  Firebird -> Return [order 6] : [FA!=0]
  El_Dorado -> Return [order 6] : [FA!=0]
  Firebird -> Return [order 4] : [(EnblSOCTerm==1) && (SOC<(SOCDeplete))]
  Firebird -> Return [order 1] : [Run==0]
  Firebird -> Return [order 2] : [(LoopTime>= ProfileEndTime) && (LoopTime>0)]
  Firebird -> Return [order 3] : [SkipStep==1]
  Regal -> Return [order 6] : [FA!=0]
  El_Dorado -> Return [order 4] : [SwitchMode==1]
  Regal -> Return [order 4] : [(EnblSOCTerm==1) && (SOC<(SOCDeplete))]
  Regal -> Return [order 1] : [Run==0]
  Regal -> Return [order 2] : [(LoopTime>= ProfileEndTime) && (LoopTime>0)]
  Regal -> Return [order 3] : [SkipStep==1]
  Silverado -> Return [order 6] : [FA!=0]
  ELR -> Return [order 5] : [SwitchMode==1]
  Silverado -> Return [order 4] : [(EnblSOCTerm==1) && (SOC<(SOCDeplete))]
  Silverado -> Return [order 1] : [Run==0]
  Silverado -> Return [order 2] : [(LoopTime>= ProfileEndTime) && (LoopTime>0)]
  Silverado -> Return [order 3] : [SkipStep==1]
  Sierra -> Return [order 5] : [FA!=0]
  Determine_Idle_Type -> Determine_Idle_ConstPower_Time [order 1] : [ProfileTypeIndex == 1]
  Sierra -> Return [order 4] : [(EnblSOCTerm==1) && (SOC<(SOCDeplete))]
  Sierra -> Return [order 1] : [Run==0]
  Sierra -> Return [order 2] : [(LoopTime>= ProfileEndTime) && (LoopTime>0)]
  Sierra -> Return [order 3] : [SkipStep==1]
  Sonic -> Return [order 5] : [FA!=0]
  Determine_Idle_Type -> Determine_Idle_ConstCurrent_Time [order 2] : [ProfileTypeIndex == 2]
  Sonic -> Return [order 4] : [(EnblSOCTerm==1) && (SOC<(SOCDeplete))]
  Sonic -> Return [order 1] : [Run==0]
  Sonic -> Return [order 2] : [(LoopTime>= ProfileEndTime) && (LoopTime>0)]
  Sonic -> Return [order 3] : [SkipStep==1]
  Spark -> Return [order 5] : [FA!=0]
  Determine_IdleCurrent -> Return [order 2] : [(CurrentReq)==0 && (ManualIdle!=1)]
  Spark -> Return [order 4] : [(EnblSOCTerm==1) && (SOC<(SOCDeplete))]
  Spark -> Return [order 1] : [Run==0]
  Spark -> Return [order 2] : [(LoopTime>= ProfileEndTime) && (LoopTime>0)]
  Spark -> Return [order 3] : [SkipStep==1]
  Sky -> Return [order 5] : [FA!=0]
  Determine_IdleCurrent -> Idle_ConstCurrent [order 1] : [(CurrentReq!=0) || (ManualIdle==1)]
  Sky -> Return [order 4] : [(EnblSOCTerm==1) && (SOC<(SOCDeplete))]
  Sky -> Return [order 1] : [Run==0]
  Sky -> Return [order 2] : [(LoopTime>= ProfileEndTime) && (LoopTime>0)]
  Sky -> Return [order 3] : [SkipStep==1]
  Solstice -> Return [order 6] : [FA!=0]
  Solstice -> Return [order 5] : [SwitchMode==1]
  Solstice -> Return [order 4] : [(EnblSOCTerm==1) && (SOC<(SOCDeplete))]
  Solstice -> Return [order 1] : [Run==0]
  Solstice -> Return [order 2] : [(LoopTime>= ProfileEndTime) && (LoopTime>0)]
  Solstice -> Return [order 3] : [SkipStep==1]
  SRX -> Return [order 6] : [FA!=0]
  SRX -> Return [order 5] : [SwitchMode==1]
  SRX -> Return [order 4] : [(EnblSOCTerm==1) && (SOC<(SOCDeplete))]
  SRX -> Return [order 1] : [Run==0]
  SRX -> Return [order 2] : [(LoopTime>= ProfileEndTime) && (LoopTime>0)]
  SRX -> Return [order 3] : [SkipStep==1]
  Escalade -> Return [order 6] : [FA!=0]
  Escalade -> Return [order 5] : [SwitchMode==1]
  Escalade -> Return [order 4] : [(EnblSOCTerm==1) && (SOC<(SOCDeplete))]
  Escalade -> Return [order 1] : [Run==0]
  Escalade -> Return [order 2] : [(LoopTime>= ProfileEndTime) && (LoopTime>0)]
  Escalade -> Return [order 3] : [SkipStep==1]
  Terrain -> Return [order 6] : [FA!=0]
  Terrain -> Return [order 5] : [SwitchMode==1]
  Terrain -> Return [order 4] : [(EnblSOCTerm==1) && (SOC<(SOCDeplete))]
  Terrain -> Return [order 1] : [Run==0]
  Terrain -> Return [order 2] : [(LoopTime>= ProfileEndTime) && (LoopTime>0)]
  Terrain -> Return [order 3] : [SkipStep==1]
  Torrent -> Return [order 6] : [FA!=0]
  Torrent -> Return [order 5] : [SwitchMode==1]
  Torrent -> Return [order 4] : [(EnblSOCTerm==1) && (SOC<(SOCDeplete))]
  Torrent -> Return [order 1] : [Run==0]
  Torrent -> Return [order 2] : [(LoopTime>= ProfileEndTime) && (LoopTime>0)]
  Torrent -> Return [order 3] : [SkipStep==1]
  TransAm -> Return [order 6] : [FA!=0]
  TransAm -> Return [order 5] : [SwitchMode==1]
  TransAm -> Return [order 4] : [(EnblSOCTerm==1) && (SOC<(SOCDeplete))]
  TransAm -> Return [order 1] : [Run==0]
  TransAm -> Return [order 2] : [(LoopTime>= ProfileEndTime) && (LoopTime>0)]
  TransAm -> Return [order 3] : [SkipStep==1]
  Traverse -> Return [order 6] : [FA!=0]
  Traverse -> Return [order 5] : [SwitchMode==1]
  Traverse -> Return [order 4] : [(EnblSOCTerm==1) && (SOC<(SOCDeplete))]
  Traverse -> Return [order 1] : [Run==0]
  Traverse -> Return [order 2] : [(LoopTime>= ProfileEndTime) && (LoopTime>0)]
  Traverse -> Return [order 3] : [SkipStep==1]
  Tahoe -> Return [order 6] : [FA!=0]
  Tahoe -> Return [order 5] : [SwitchMode==1]
  Tahoe -> Return [order 4] : [(EnblSOCTerm==1) && (SOC<(SOCDeplete))]
  Tahoe -> Return [order 1] : [Run==0]
  Tahoe -> Return [order 2] : [(LoopTime>= ProfileEndTime) && (LoopTime>0)]
  Tahoe -> Return [order 3] : [SkipStep==1]
  Verano -> Return [order 6] : [FA!=0]
  Verano -> Return [order 5] : [SwitchMode==1]
  Verano -> Return [order 4] : [(EnblSOCTerm==1) && (SOC<(SOCDeplete))]
  Verano -> Return [order 1] : [Run==0]
  Verano -> Return [order 2] : [(LoopTime>= ProfileEndTime) && (LoopTime>0)]
  Verano -> Return [order 3] : [SkipStep==1]
  XTS -> Return [order 6] : [FA!=0]
  XTS -> Return [order 5] : [SwitchMode==1]
  XTS -> Return [order 4] : [(EnblSOCTerm==1) && (SOC<(SOCDeplete))]
  XTS -> Return [order 1] : [Run==0]
  XTS -> Return [order 2] : [(LoopTime>= ProfileEndTime) && (LoopTime>0)]
  XTS -> Return [order 3] : [SkipStep==1]
  Yukon -> Return [order 6] : [FA!=0]
  Yukon -> Return [order 5] : [SwitchMode==1]
  Yukon -> Return [order 4] : [(EnblSOCTerm==1) && (SOC<(SOCDeplete))]
  Yukon -> Return [order 1] : [Run==0]
  Yukon -> Return [order 2] : [(LoopTime>= ProfileEndTime) && (LoopTime>0)]
  Yukon -> Return [order 3] : [SkipStep==1]
  Determine_SetChamberT_ToBatTemp -> Apply_SetChamberT_ToBatTemp [order 1] : [SetChamberT_ToBatTemp != 0]
  SwitchProfile -> Determine_Idle_Type [order 11] : [ProfileClassIndex==8]
  SwitchProfile -> Increment_Test [order 15] : [ProfileClassIndex == 18]
  SwitchProfile -> Determine_CurrentLimit [order 14] : [ProfileClassIndex == 10]
  SwitchProfile -> OCV_Test [order 9] : [ProfileClassIndex==9]
  Idle_ConstCurrent -> Return [order 4] : [SkipStep==1]
  Idle_ConstCurrent -> Return [order 3] : [(IdleStep==99) && (Wait>1)]
  Idle_ConstCurrent -> Return [order 1] : [Run==0]
  Determine_Idle_ConstCurrent_Time -> Determine_IdleCurrent [order 1] : [IdleTime!=0]
  Determine_Idle_ConstCurrent_Time -> Return [order 2] : [IdleTime==0]
  Idle_ConstCurrent -> Return [order 2] : [FA!=0]
  Firebird -> Return [order 5] : [SwitchMode==1]
  Regal -> Return [order 5] : [SwitchMode==1]
  Silverado -> Return [order 5] : [SwitchMode==1]
  SwitchProfile -> Repeat [order 3] : [ProfileClassIndex==100&&RepeatIndex==0]
  RepeatEnd -> SwitchProfile
  Repeat -> RepeatJumpLoop
  RepeatJumpLoop -> RepeatEnd [order 2] : [RepeatIndex == (RepeatCount+1)]
  RepeatJumpLoop -> SwitchProfile [order 1] : [RepeatIndex != (RepeatCount+1)]
  Return -> start [order 2] : [Run == 0]
  data: ProfileList function_input uint8 size=20; index function_input double; ProfileInd function_output uint8 size=1; ProfileList function_input uint8 size=20; index function_input double; ProfileInd function_output uint8 size=1; ProfileList function_input uint8 size=20; index function_input double; ProfileInd function_output uint8 size=1; ProfileList function_input uint8 size=20; index function_input double; ProfileInd function_output uint8 size=1; ProfileList function_input double size=20; index function_input double; ProfileInd function_output double size=1; ProfileList function_input double size=20; index function_input double; ProfileInd function_output double size=1; SuiteList function_input uint8 size=12; index function_input uint8; ProfileInd function_output uint8 size=1; ProfileList function_input double size=20; index function_input double; ProfileInd function_output double size=1; ProfileList function_input double size=20; index function_input double; ProfileInd function_output double size=1; ProfileList function_input double size=20; index function_input double; ProfileInd function_output double size=1; ProfileList function_input double size=20; index function_input double; ProfileInd function_output double size=1; ProfileList function_input double size=20; index function_input double; ProfileInd function_output double size=1; ProfileList function_input double size=20; index function_input double; ProfileInd function_output double size=1; ProfileList function_input double size=20; index function_input double; ProfileInd function_output double size=1; ProfileList function_input uint8 size=20; index function_input double; ProfileInd function_output uint8 size=1; ProfileList function_input double size=20; index function_input double; ProfileInd function_output double size=1; ProfileList function_input double size=20; index function_input double; ProfileInd function_output double size=1; ProfileList function_input double size=20; index function_input double; ProfileInd function_output double size=1; ProfileList function_input double size=20; index function_input double; ProfileInd function_output double size=1; ProfileList function_input double size=20; index function_input double; ProfileInd function_output double size=1; ProfileList function_input uint8 size=20; index function_input double; ProfileInd function_output uint8 size=1; Jumps local int8; RepeatCount local int8; data local double; ProfileList function_input double size=20; index function_input double; ProfileInd function_output double size=1; Jumps local int8; RepeatCount local int8; ProfileList function_input double size=20; index function_input double; ProfileInd function_output double size=1; ProfileEndTime input double; SOC input double; VoltTarget output double; PowerCycle output double; LoopTime input single; IndicatorSF output double; ChargeCurrSelect output single; ChargeStep input double; sim_step_time input double; Direction output single; PulseStep input single; ManualMode input double; RestTimeIn input double; RestTime local double; Run input boolean; SuiteSchedule input uint8 size=12; Wait local double; ProfileScheduleClassIn input uint8 size=20; i local single; ProfileClassIndex local uint8 size=1; ResetSOC output boolean; ResetWaitTime local double; ProfileScheduleTypeIn input uint8 size=20; ProfileScheduleParameterIn input double size=20; ProfileScheduleParameterIn2 input double size=20; SkipStep input boolean; ProfileTypeIndex local uint8 size=1; ProfileParameter local double; RestTimeTarget local double; SuiteStep output uint8; ProfileScheduleClass output uint8 size=20; ProfileScheduleType output uint8 size=20; ProfileScheduleParameter output double size=20; Step output single; Suite output single; SuiteIndex local uint8; PrimePackClass local uint8 size=20 =1 5 4 1 1 5 0 0 0 0 0 0 0 0 0 0 0 0 0 0; PrimePackType local uint8 size=20 =4 0 0 5 5 0 0 0 0 0 0 0 0 0 0 0 0 0 0 0; PrimePackParameter local double size=20 =0 3600 0 80 94 0 3600 0 0 0 0 0 0 0 0 0 0 0 0 0; DrivesWithPulsesClass local uint8 size=20 =2 2 3 2 3 2 0 0 0 0 0 0 0 0 0 0 0 0 0 0; DrivesWithPulsesType local uint8 size=20 =1 4 1 2 2 2 0 0 0 0 0 0 0 0 0 0 0 0 0 0; DrivesWithPulsesParameter local double size=20 =0 0 0 0 0 0 0 0 0 0 0 0 0 0 0 0 0 0 0 0; DriveToPICClass local uint8 size=20 =2 2 2 5 1 5 0 0 0 0 0 0 0 0 0 0 0 0 0 0; DriveToPICType local uint8 size=20 =1 4 2 0 1 0 0 0 0 0 0 0 0 0 0 0 0 0 0 0; DriveToPICParameter local double size=20 =0 0 0 3600 0 3600 0 0 0 0 0 0 0 0 0 0 0 0 0 0; EnblSOCTerm input boolean; SOCDeplete input single; DriveToPICClass_Init local double; DriveToPICParameter_Init local double; DriveToPICType_Init local double; DrivesWithPulsesClass_Init local double; DrivesWithPulsesParameter_Init local double; DrivesWithPulsesType_Init local double; PrimePackClass_Init local double; PrimePackParameter_Init local double; PrimePackType_Init local double; ResetTarget local double; ResetTime local double; ResetRun output double; CapStep input single; WTime local double; EndStep output double; OCVStep input single; SOCTarget output double; SwitchMode input double; StartTime output double; EndTime output double; ProfileScheduleParameter2 local double size=20; FA input double; IdleStep input double; IdleTime output double; PowerReq output double; CurrentReq output double; ManualIdle input double; Rate output single; CurrLim output double; RateStep input double; IncrementStep input double; SetChamberT_ToBatTemp output boolean; RepeatIndex local double; Idle_Type output double; RepeatStep local double; data1 local double; Jumps local double; RepeatCount local double
  function ProfileInd  = GetIndex(ProfileList,index):
    | function ProfileInd  = GetIndex(ProfileList,index)
    | 
    | ProfileInd = ProfileList(index);
    | 
    | end
  function ProfileInd  = GetIndex(ProfileList,index):
    | function ProfileInd  = GetIndex(ProfileList,index)
    | 
    | ProfileInd = ProfileList(index);
    | 
    | end
  function ProfileInd  = GetIndex(ProfileList,index):
    | function ProfileInd  = GetIndex(ProfileList,index)
    | 
    | ProfileInd = ProfileList(index);
    | 
    | end
  function ProfileInd  = GetIndex(ProfileList,index):
    | function ProfileInd  = GetIndex(ProfileList,index)
    | 
    | ProfileInd = ProfileList(index);
    | 
    | end
  function ProfileInd  = GetIndex(ProfileList,index):
    | function ProfileInd  = GetIndex(ProfileList,index)
    | 
    | ProfileInd = ProfileList(index);
    | 
    | end
  function ProfileInd  = GetIndex(ProfileList,index):
    | function ProfileInd  = GetIndex(ProfileList,index)
    | 
    | ProfileInd = ProfileList(index);
    | 
    | end
  function ProfileInd  = GetSuiteIndex(SuiteList,index):
    | function ProfileInd  = GetSuiteIndex(SuiteList,index)
    | 
    | ProfileInd = SuiteList(index);
    | 
    | end
  function ProfileInd  = GetIndex(ProfileList,index):
    | function ProfileInd  = GetIndex(ProfileList,index)
    | 
    | ProfileInd = ProfileList(index);
    | 
    | end
  function ProfileInd  = GetIndex(ProfileList,index):
    | function ProfileInd  = GetIndex(ProfileList,index)
    | 
    | ProfileInd = ProfileList(index);
    | 
    | end
  function ProfileInd  = GetIndex(ProfileList,index):
    | function ProfileInd  = GetIndex(ProfileList,index)
    | 
    | ProfileInd = ProfileList(index);
    | 
    | end
  function ProfileInd  = GetIndex(ProfileList,index):
    | function ProfileInd  = GetIndex(ProfileList,index)
    | 
    | ProfileInd = ProfileList(index);
    | 
    | end
  function ProfileInd  = GetIndex(ProfileList,index):
    | function ProfileInd  = GetIndex(ProfileList,index)
    | 
    | ProfileInd = ProfileList(index);
    | 
    | end
  function ProfileInd  = GetIndex(ProfileList,index):
    | function ProfileInd  = GetIndex(ProfileList,index)
    | 
    | ProfileInd = ProfileList(index);
    | 
    | end
  function ProfileInd  = GetIndex(ProfileList,index):
    | function ProfileInd  = GetIndex(ProfileList,index)
    | 
    | ProfileInd = ProfileList(index);
    | 
    | end
  function ProfileInd  = GetIndex(ProfileList,index):
    | function ProfileInd  = GetIndex(ProfileList,index)
    | 
    | ProfileInd = ProfileList(index);
    | 
    | end
  function ProfileInd  = GetIndex(ProfileList,index):
    | function ProfileInd  = GetIndex(ProfileList,index)
    | 
    | ProfileInd = ProfileList(index);
    | 
    | end
  function ProfileInd  = GetIndex(ProfileList,index):
    | function ProfileInd  = GetIndex(ProfileList,index)
    | 
    | ProfileInd = ProfileList(index);
    | 
    | end
  function ProfileInd  = GetIndex(ProfileList,index):
    | function ProfileInd  = GetIndex(ProfileList,index)
    | 
    | ProfileInd = ProfileList(index);
    | 
    | end
  function ProfileInd  = GetIndex(ProfileList,index):
    | function ProfileInd  = GetIndex(ProfileList,index)
    | 
    | ProfileInd = ProfileList(index);
    | 
    | end
  function ProfileInd  = GetIndex(ProfileList,index):
    | function ProfileInd  = GetIndex(ProfileList,index)
    | 
    | ProfileInd = ProfileList(index);
    | 
    | end
  function ProfileInd  = GetIndex(ProfileList,index):
    | function ProfileInd  = GetIndex(ProfileList,index)
    | 
    | ProfileInd = ProfileList(index);
    | 
    | end
  function ProfileInd  = GetIndex(ProfileList,index):
    | function ProfileInd  = GetIndex(ProfileList,index)
    | 
    | ProfileInd = ProfileList(index);
    | 
    | end
  function ProfileInd  = GetIndex(ProfileList,index):
    | function ProfileInd  = GetIndex(ProfileList,index)
    | 
    | ProfileInd = ProfileList(index);
    | 
    | end
